simulink model "planning_control"  (R2020a)
settings: Solver=VariableStepAuto  StartTime=0.0  StopTime=40  RelTol=1e-3
undefined symbols (not defined in the file): aubr, tablebr, vubr
libraries: simulink x6, Solver_SF x2
settings Model: Creator=czj  LastModifiedBy=czj

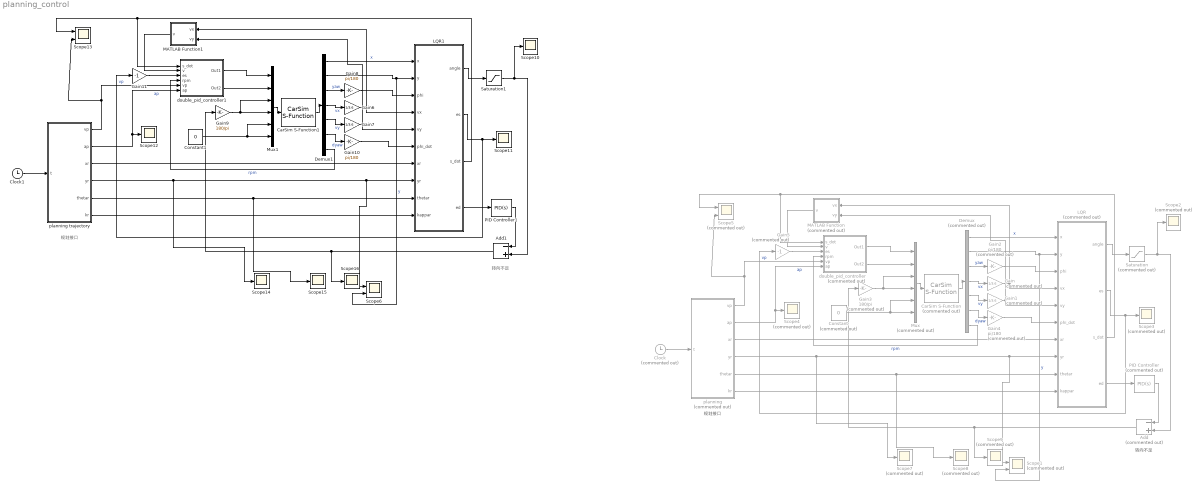
== system planning_control ==
  note: 规划接口
  note: 转向不足
  note: 规划接口
  note: 转向不足
  Add : Sum  Commented=on  Inputs=-+
  Add1 : Sum  Inputs=-+
  CarSim S-Function : Solver_SF/CarSim S-Function  Priority=1  Commented=on  SIMFILE=simfile.sim  Run_RTs=off  vs_state_ind=Run  StopMode_ind=Vehicle Model
  CarSim S-Function1 : Solver_SF/CarSim S-Function  Priority=1  SIMFILE=simfile.sim  Run_RTs=off  vs_state_ind=Run  StopMode_ind=Vehicle Model
  Clock : Clock  Commented=on
  Clock1 : Clock
  Constant : Constant  Commented=on  Value=0
  Constant1 : Constant  Value=0
  Demux : Demux  Commented=on  Outputs=7
  Demux1 : Demux  Outputs=7
  Gain : Gain  Commented=on  Gain=1/3.6
  Gain1 : Gain  Commented=on  Gain=1/3.6
  Gain10 : Gain  Gain=pi/180
  Gain11 : Gain  Gain=-1
  Gain2 : Gain  Commented=on  Gain=pi/180
  Gain3 : Gain  Commented=on  Gain=180/pi
  Gain4 : Gain  Commented=on  Gain=pi/180
  Gain5 : Gain  Commented=on  Gain=-1
  Gain6 : Gain  Gain=1/3.6
  Gain7 : Gain  Gain=1/3.6
  Gain8 : Gain  Gain=pi/180
  Gain9 : Gain  Gain=180/pi
  LQR : Subsystem  Commented=on
  LQR1 : Subsystem
  MATLAB Function : MATLAB Function  Commented=on  TreatAsAtomicUnit=on
  MATLAB Function1 : MATLAB Function  TreatAsAtomicUnit=on
  Mux : Mux  Commented=on  Inputs=6
  Mux1 : Mux  Inputs=6
  PID Controller : simulink/Continuous/PID Controller  Commented=on  Controller=PID  Form=Parallel  TimeDomain=Continuous-time  UseExternalTs=off  SampleTime=-1  IntegratorMethod=Forward Euler  FilterMethod=Forward Euler  ControllerParametersSource=internal  P=0  I=0  D=0  UseFilter=on  N=100  TunerSelectOption=Transfer Function Based (PID Tuner App)  InitialConditionSource=internal  InitialConditionForIntegrator=0  InitialConditionForFilter=0  DifferentiatorICPrevScaledInput=0  ExternalReset=none  TrackingMode=off  Kt=1  LimitOutput=off  UpperSaturationLimit=inf  LowerSaturationLimit=-inf  LinearizeAsGain=on  AntiWindupMode=none  Kb=1  POutMin=[]  POutMax=[]  IOutMin=[]  IOutMax=[]  DOutMin=[]  DOutMax=[]  NOutMin=[]  NOutMax=[]  SumOutMin=[]  SumOutMax=[]  SaturationOutMin=[]  SaturationOutMax=[]  PParamMin=[]  PParamMax=[]  IParamMin=[]  IParamMax=[]  DParamMin=[]  DParamMax=[]  NParamMin=[]  NParamMax=[]  KbParamMin=[]  KbParamMax=[]  KtParamMin=[]  KtParamMax=[]  KbOutMin=[]  KbOutMax=[]  KtOutMin=[]  KtOutMax=[]  IntegratorOutMin=[]  IntegratorOutMax=[]  FilterOutMin=[]  FilterOutMax=[]  SumI1OutMin=[]  SumI1OutMax=[]  SumI2OutMin=[]  SumI2OutMax=[]  SumI3OutMin=[]  SumI3OutMax=[]  SumI4OutMin=[]  SumI4OutMax=[]  SumDOutMin=[]  SumDOutMax=[]  DifferentiatorOutMin=[]  DifferentiatorOutMax=[]  FilterDiffOutCoefMin=[]  FilterDiffOutCoefMax=[]  ReciprocalOutMin=[]  ReciprocalOutMax=[]  SumDenOutMin=[]  SumDenOutMax=[]  SumNumOutMin=[]  SumNumOutMax=[]  DivideOutMin=[]  DivideOutMax=[]  UdiffTsProdOutMin=[]  UdiffTsProdOutMax=[]  NTsProdOutMin=[]  NTsProdOutMax=[]  UintegralTsProdOutMin=[]  UintegralTsProdOutMax=[]  UngainTsProdOutMin=[]  UngainTsProdOutMax=[]  IntegratorContinuousStateAttributes=''  IntegratorStateMustResolveToSignalObject=off  IntegratorRTWStateStorageClass=Auto  FilterContinuousStateAttributes=''  FilterStateMustResolveToSignalObject=off  FilterRTWStateStorageClass=Auto  ParallelPVariant=InternalParameters  IdealPVariant=Disabled  IVariant=InternalParameters  DVariant=InternalParameters  IntegratorVariant=Continuous  SatVariant=Disabled  AWVariant=Passthrough  PCopyVariant=Disabled  TRVariant=Disabled  FdbkBlocksVariant=Forward  IdealPFdbkVariant=Disabled  SatFdbkVariant=Disabled  DerivativeFilterVariant=ContFilter  NVariant=InternalParameters  NCopyVariant=Disabled  FilterICVariant=InternalICsFilter  IntegratorICVariant=InternalICs  ExternalResetVariant=Disabled  TRSumVariant=Passthrough  SumFdbkVariant=Disabled  SumVariant=Sum_PID  TsampFilterVariant=InternalTs  TsampNgainVariant=Passthrough  TsampIntegralVariant=Passthrough
  PID Controller1 : simulink/Continuous/PID Controller  Controller=PID  Form=Parallel  TimeDomain=Continuous-time  UseExternalTs=off  SampleTime=-1  IntegratorMethod=Forward Euler  FilterMethod=Forward Euler  ControllerParametersSource=internal  P=0  I=0  D=0  UseFilter=on  N=100  TunerSelectOption=Transfer Function Based (PID Tuner App)  InitialConditionSource=internal  InitialConditionForIntegrator=0  InitialConditionForFilter=0  DifferentiatorICPrevScaledInput=0  ExternalReset=none  TrackingMode=off  Kt=1  LimitOutput=off  UpperSaturationLimit=inf  LowerSaturationLimit=-inf  LinearizeAsGain=on  AntiWindupMode=none  Kb=1  POutMin=[]  POutMax=[]  IOutMin=[]  IOutMax=[]  DOutMin=[]  DOutMax=[]  NOutMin=[]  NOutMax=[]  SumOutMin=[]  SumOutMax=[]  SaturationOutMin=[]  SaturationOutMax=[]  PParamMin=[]  PParamMax=[]  IParamMin=[]  IParamMax=[]  DParamMin=[]  DParamMax=[]  NParamMin=[]  NParamMax=[]  KbParamMin=[]  KbParamMax=[]  KtParamMin=[]  KtParamMax=[]  KbOutMin=[]  KbOutMax=[]  KtOutMin=[]  KtOutMax=[]  IntegratorOutMin=[]  IntegratorOutMax=[]  FilterOutMin=[]  FilterOutMax=[]  SumI1OutMin=[]  SumI1OutMax=[]  SumI2OutMin=[]  SumI2OutMax=[]  SumI3OutMin=[]  SumI3OutMax=[]  SumI4OutMin=[]  SumI4OutMax=[]  SumDOutMin=[]  SumDOutMax=[]  DifferentiatorOutMin=[]  DifferentiatorOutMax=[]  FilterDiffOutCoefMin=[]  FilterDiffOutCoefMax=[]  ReciprocalOutMin=[]  ReciprocalOutMax=[]  SumDenOutMin=[]  SumDenOutMax=[]  SumNumOutMin=[]  SumNumOutMax=[]  DivideOutMin=[]  DivideOutMax=[]  UdiffTsProdOutMin=[]  UdiffTsProdOutMax=[]  NTsProdOutMin=[]  NTsProdOutMax=[]  UintegralTsProdOutMin=[]  UintegralTsProdOutMax=[]  UngainTsProdOutMin=[]  UngainTsProdOutMax=[]  IntegratorContinuousStateAttributes=''  IntegratorStateMustResolveToSignalObject=off  IntegratorRTWStateStorageClass=Auto  FilterContinuousStateAttributes=''  FilterStateMustResolveToSignalObject=off  FilterRTWStateStorageClass=Auto  ParallelPVariant=InternalParameters  IdealPVariant=Disabled  IVariant=InternalParameters  DVariant=InternalParameters  IntegratorVariant=Continuous  SatVariant=Disabled  AWVariant=Passthrough  PCopyVariant=Disabled  TRVariant=Disabled  FdbkBlocksVariant=Forward  IdealPFdbkVariant=Disabled  SatFdbkVariant=Disabled  DerivativeFilterVariant=ContFilter  NVariant=InternalParameters  NCopyVariant=Disabled  FilterICVariant=InternalICsFilter  IntegratorICVariant=InternalICs  ExternalResetVariant=Disabled  TRSumVariant=Passthrough  SumFdbkVariant=Disabled  SumVariant=Sum_PID  TsampFilterVariant=InternalTs  TsampNgainVariant=Passthrough  TsampIntegralVariant=Passthrough
  Saturation : Saturate  Commented=on  UpperLimit=1  LowerLimit=-1
  Saturation1 : Saturate  UpperLimit=1  LowerLimit=-1
  Scope1 : Scope  Commented=on  NumInputPorts=2
  Scope{10..12,14..16} (6 alike) : Scope
  Scope13 : Scope  NumInputPorts=2
  Scope{2..4,7..9} (6 alike) : Scope  Commented=on
  Scope5 : Scope  Commented=on  NumInputPorts=2
  Scope6 : Scope  NumInputPorts=2
  double_pid_controller : Subsystem  Commented=on
  double_pid_controller1 : Subsystem
  planning : MATLAB Function  Commented=on  TreatAsAtomicUnit=on
  planning trajectory : MATLAB Function  TreatAsAtomicUnit=on
  wires:
  CarSim S-Function/1 -> Demux/1
  PID Controller/1 -> Add/1
  LQR/3(s_dot) -> double_pid_controller/1(s_dot), Scope5/1
  Add/1 -> Scope9/1, Gain3/1
  Gain3/1 -> Mux/4, Mux/3
  Saturation/1 -> Scope2/1, Add/2
  planning/6(kr) -> LQR/10(kappar)
  LQR/2(es) -> Scope3/1, Gain5/1
  LQR/4(ed) -> PID Controller/1
  double_pid_controller/2(Out2) -> Mux/2
  Constant/1 -> Mux/5, Mux/6
  planning/2(ap) -> Scope4/1, double_pid_controller/6(ap)  "ap"
  Demux/3 -> Gain2/1  "yaw"
  Gain/1 -> MATLAB Function/1(vx), LQR/4(vx)
  Gain4/1 -> LQR/6(phi_dot)
  planning/3(xr) -> LQR/7(xr)
  Demux/6 -> Gain4/1  "dyaw"
  Mux/1 -> CarSim S-Function/1
  Gain5/1 -> double_pid_controller/3(es)
  Demux/5 -> Gain1/1  "vy"
  Demux/2 -> Scope1/2, LQR/2(y)  "y"
  double_pid_controller/1(Out1) -> Mux/1
  planning/5(thetar) -> Scope8/1, LQR/9(thetar)
  LQR/1(angle) -> Saturation/1
  planning/1(vp) -> Scope5/2, double_pid_controller/5(vp)  "vp"
  Gain1/1 -> MATLAB Function/2(vy), LQR/5(vy)
  Demux/7 -> double_pid_controller/4(rpm)  "rpm"
  Demux/1 -> LQR/1(x)  "x"
  Clock/1 -> planning/1(t)
  planning/4(yr) -> Scope7/1, Scope1/1, LQR/8(yr)
  MATLAB Function/1(v) -> double_pid_controller/2(v)
  Demux/4 -> Gain/1  "vx"
  Gain2/1 -> LQR/3(phi)
  CarSim S-Function1/1 -> Demux1/1
  PID Controller1/1 -> Add1/1
  LQR1/3(s_dot) -> double_pid_controller1/1(s_dot), Scope13/1
  Add1/1 -> Scope16/1, Gain9/1
  Gain9/1 -> Mux1/4, Mux1/3
  Saturation1/1 -> Scope10/1, Add1/2
  planning trajectory/6(kr) -> LQR1/10(kappar)
  LQR1/2(es) -> Scope11/1, Gain11/1
  LQR1/4(ed) -> PID Controller1/1
  double_pid_controller1/2(Out2) -> Mux1/2
  Constant1/1 -> Mux1/5, Mux1/6
  planning trajectory/2(ap) -> Scope12/1, double_pid_controller1/6(ap)  "ap"
  Demux1/3 -> Gain8/1  "yaw"
  Gain6/1 -> MATLAB Function1/1(vx), LQR1/4(vx)
  Gain10/1 -> LQR1/6(phi_dot)
  planning trajectory/3(xr) -> LQR1/7(xr)
  Demux1/6 -> Gain10/1  "dyaw"
  Mux1/1 -> CarSim S-Function1/1
  Gain11/1 -> double_pid_controller1/3(es)
  Demux1/5 -> Gain7/1  "vy"
  Demux1/2 -> Scope6/2, LQR1/2(y)  "y"
  double_pid_controller1/1(Out1) -> Mux1/1
  planning trajectory/5(thetar) -> Scope15/1, LQR1/9(thetar)
  LQR1/1(angle) -> Saturation1/1
  planning trajectory/1(vp) -> Scope13/2, double_pid_controller1/5(vp)  "vp"
  Gain7/1 -> MATLAB Function1/2(vy), LQR1/5(vy)
  Demux1/7 -> double_pid_controller1/4(rpm)  "rpm"
  Demux1/1 -> LQR1/1(x)  "x"
  Clock1/1 -> planning trajectory/1(t)
  planning trajectory/4(yr) -> Scope14/1, Scope6/1, LQR1/8(yr)
  MATLAB Function1/1(v) -> double_pid_controller1/2(v)
  Demux1/4 -> Gain6/1  "vx"
  Gain8/1 -> LQR1/3(phi)

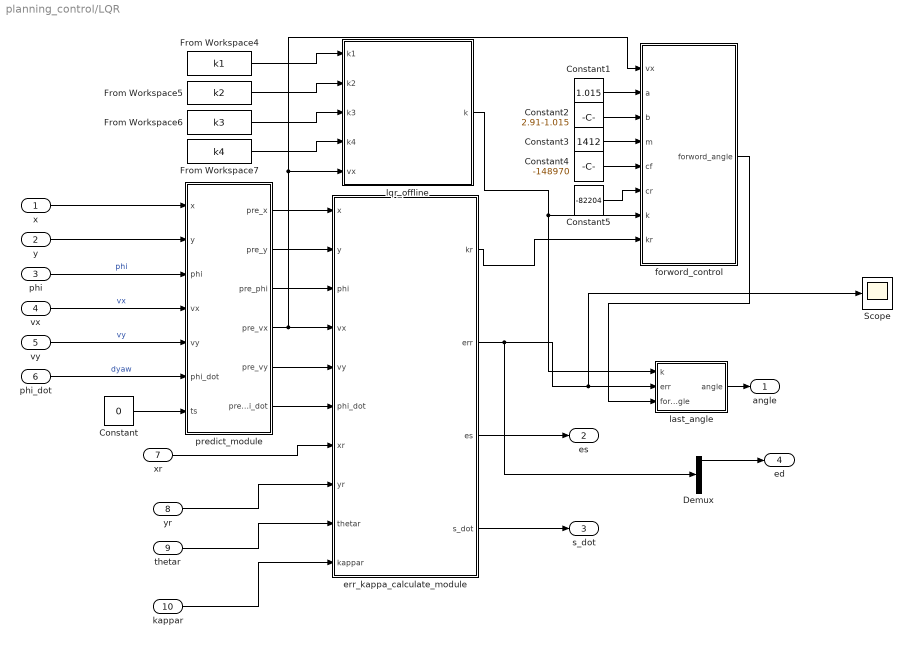
== system planning_control/LQR ==
  x : Inport
  y : Inport  Port=2
  phi : Inport  Port=3
  vx : Inport  Port=4
  vy : Inport  Port=5
  phi_dot : Inport  Port=6
  xr : Inport  Port=7
  yr : Inport  Port=8
  thetar : Inport  Port=9
  kappar : Inport  Port=10
  Constant : Constant  Value=0
  Constant1 : Constant  Value=1.015
  Constant2 : Constant  Value=2.91-1.015
  Constant3 : Constant  Value=1412
  Constant4 : Constant  Value=-148970
  Constant5 : Constant  Value=-82204
  Demux : Demux
  From Workspace4 : FromWorkspace  VariableName=k1
  From Workspace5 : FromWorkspace  VariableName=k2
  From Workspace6 : FromWorkspace  VariableName=k3
  From Workspace7 : FromWorkspace  VariableName=k4
  Scope : Scope
  err_kappa_calculate_module : MATLAB Function  TreatAsAtomicUnit=on
  forword_control : MATLAB Function  TreatAsAtomicUnit=on
  last_angle : MATLAB Function  TreatAsAtomicUnit=on
  lqr_offline : MATLAB Function  TreatAsAtomicUnit=on
  predict_module : MATLAB Function  TreatAsAtomicUnit=on
  angle : Outport  VectorParamsAs1DForOutWhenUnconnected=off
  es : Outport  Port=2  VectorParamsAs1DForOutWhenUnconnected=off
  s_dot : Outport  Port=3  VectorParamsAs1DForOutWhenUnconnected=off
  ed : Outport  Port=4  VectorParamsAs1DForOutWhenUnconnected=off
  wires:
  From Workspace7/1 -> lqr_offline/4(k4)
  vy/1 -> predict_module/5(vy)  "vy"
  From Workspace6/1 -> lqr_offline/3(k3)
  x/1 -> predict_module/1(x)
  lqr_offline/1(k) -> last_angle/1(k), forword_control/7(k)
  predict_module/2(pre_y) -> err_kappa_calculate_module/2(y)
  err_kappa_calculate_module/1(kr) -> forword_control/8(kr)
  forword_control/1(forword_angle) -> last_angle/3(forword_angle)
  predict_module/4(pre_vx) -> lqr_offline/5(vx), forword_control/1(vx), err_kappa_calculate_module/4(vx)
  phi_dot/1 -> predict_module/6(phi_dot)  "dyaw"
  last_angle/1(angle) -> angle/1
  From Workspace5/1 -> lqr_offline/2(k2)
  vx/1 -> predict_module/4(vx)  "vx"
  y/1 -> predict_module/2(y)
  phi/1 -> predict_module/3(phi)  "phi"
  Constant/1 -> predict_module/7(ts)
  From Workspace4/1 -> lqr_offline/1(k1)
  predict_module/1(pre_x) -> err_kappa_calculate_module/1(x)
  predict_module/5(pre_vy) -> err_kappa_calculate_module/5(vy)
  predict_module/6(pre_phi_dot) -> err_kappa_calculate_module/6(phi_dot)
  predict_module/3(pre_phi) -> err_kappa_calculate_module/3(phi)
  Constant1/1 -> forword_control/2(a)
  Constant2/1 -> forword_control/3(b)
  Constant3/1 -> forword_control/4(m)
  Constant4/1 -> forword_control/5(cf)
  xr/1 -> err_kappa_calculate_module/7(xr)
  yr/1 -> err_kappa_calculate_module/8(yr)
  thetar/1 -> err_kappa_calculate_module/9(thetar)
  kappar/1 -> err_kappa_calculate_module/10(kappar)
  err_kappa_calculate_module/3(es) -> es/1
  err_kappa_calculate_module/4(s_dot) -> s_dot/1
  Constant5/1 -> forword_control/6(cr)
  Demux/1 -> ed/1
  err_kappa_calculate_module/2(err) -> Demux/1, Scope/1, last_angle/2(err)

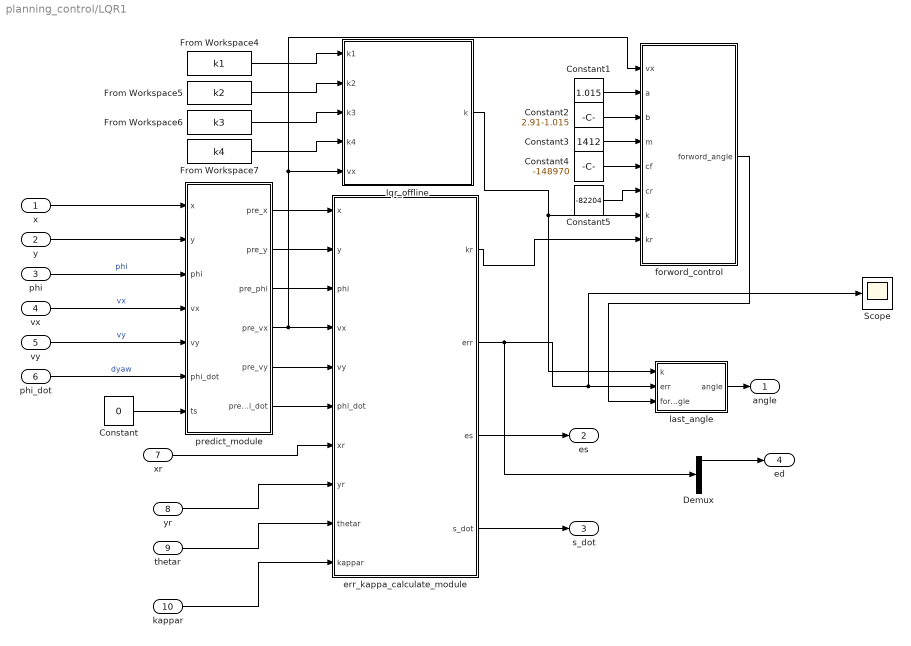
== system planning_control/LQR1 ==
  x : Inport
  y : Inport  Port=2
  phi : Inport  Port=3
  vx : Inport  Port=4
  vy : Inport  Port=5
  phi_dot : Inport  Port=6
  xr : Inport  Port=7
  yr : Inport  Port=8
  thetar : Inport  Port=9
  kappar : Inport  Port=10
  Constant : Constant  Value=0
  Constant1 : Constant  Value=1.015
  Constant2 : Constant  Value=2.91-1.015
  Constant3 : Constant  Value=1412
  Constant4 : Constant  Value=-148970
  Constant5 : Constant  Value=-82204
  Demux : Demux
  From Workspace4 : FromWorkspace  VariableName=k1
  From Workspace5 : FromWorkspace  VariableName=k2
  From Workspace6 : FromWorkspace  VariableName=k3
  From Workspace7 : FromWorkspace  VariableName=k4
  Scope : Scope
  err_kappa_calculate_module : MATLAB Function  TreatAsAtomicUnit=on
  forword_control : MATLAB Function  TreatAsAtomicUnit=on
  last_angle : MATLAB Function  TreatAsAtomicUnit=on
  lqr_offline : MATLAB Function  TreatAsAtomicUnit=on
  predict_module : MATLAB Function  TreatAsAtomicUnit=on
  angle : Outport  VectorParamsAs1DForOutWhenUnconnected=off
  es : Outport  Port=2  VectorParamsAs1DForOutWhenUnconnected=off
  s_dot : Outport  Port=3  VectorParamsAs1DForOutWhenUnconnected=off
  ed : Outport  Port=4  VectorParamsAs1DForOutWhenUnconnected=off
  wires:
  From Workspace7/1 -> lqr_offline/4(k4)
  vy/1 -> predict_module/5(vy)  "vy"
  From Workspace6/1 -> lqr_offline/3(k3)
  x/1 -> predict_module/1(x)
  lqr_offline/1(k) -> last_angle/1(k), forword_control/7(k)
  predict_module/2(pre_y) -> err_kappa_calculate_module/2(y)
  err_kappa_calculate_module/1(kr) -> forword_control/8(kr)
  forword_control/1(forword_angle) -> last_angle/3(forword_angle)
  predict_module/4(pre_vx) -> lqr_offline/5(vx), forword_control/1(vx), err_kappa_calculate_module/4(vx)
  phi_dot/1 -> predict_module/6(phi_dot)  "dyaw"
  last_angle/1(angle) -> angle/1
  From Workspace5/1 -> lqr_offline/2(k2)
  vx/1 -> predict_module/4(vx)  "vx"
  y/1 -> predict_module/2(y)
  phi/1 -> predict_module/3(phi)  "phi"
  Constant/1 -> predict_module/7(ts)
  From Workspace4/1 -> lqr_offline/1(k1)
  predict_module/1(pre_x) -> err_kappa_calculate_module/1(x)
  predict_module/5(pre_vy) -> err_kappa_calculate_module/5(vy)
  predict_module/6(pre_phi_dot) -> err_kappa_calculate_module/6(phi_dot)
  predict_module/3(pre_phi) -> err_kappa_calculate_module/3(phi)
  Constant1/1 -> forword_control/2(a)
  Constant2/1 -> forword_control/3(b)
  Constant3/1 -> forword_control/4(m)
  Constant4/1 -> forword_control/5(cf)
  xr/1 -> err_kappa_calculate_module/7(xr)
  yr/1 -> err_kappa_calculate_module/8(yr)
  thetar/1 -> err_kappa_calculate_module/9(thetar)
  kappar/1 -> err_kappa_calculate_module/10(kappar)
  err_kappa_calculate_module/3(es) -> es/1
  err_kappa_calculate_module/4(s_dot) -> s_dot/1
  Constant5/1 -> forword_control/6(cr)
  Demux/1 -> ed/1
  err_kappa_calculate_module/2(err) -> Demux/1, Scope/1, last_angle/2(err)

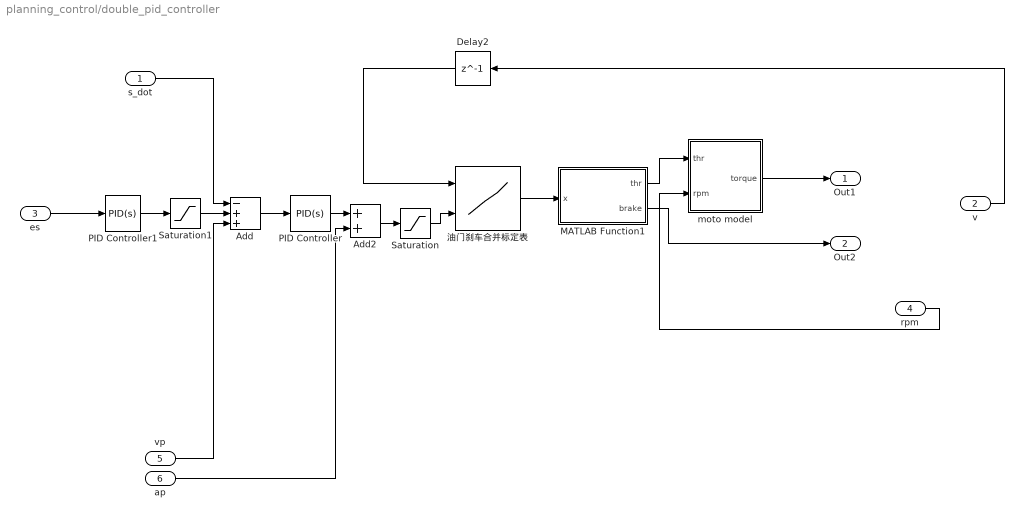
== system planning_control/double_pid_controller ==
  s_dot : Inport
  v : Inport  Port=2
  es : Inport  Port=3
  rpm : Inport  Port=4
  vp : Inport  Port=5
  ap : Inport  Port=6
  Add : Sum  Inputs=-++
  Add2 : Sum
  Delay2 : Delay  DelayLength=1
  MATLAB Function1 : MATLAB Function  TreatAsAtomicUnit=on
  PID Controller : simulink/Continuous/PID Controller  Controller=PID  Form=Parallel  TimeDomain=Continuous-time  UseExternalTs=off  SampleTime=-1  IntegratorMethod=Forward Euler  FilterMethod=Forward Euler  ControllerParametersSource=internal  P=3  I=0  D=0.1  UseFilter=on  N=30  TunerSelectOption=Transfer Function Based (PID Tuner App)  InitialConditionSource=internal  InitialConditionForIntegrator=0  InitialConditionForFilter=0  DifferentiatorICPrevScaledInput=0  ExternalReset=none  TrackingMode=off  Kt=1  LimitOutput=off  UpperSaturationLimit=inf  LowerSaturationLimit=-inf  LinearizeAsGain=on  AntiWindupMode=none  Kb=1  POutMin=[]  POutMax=[]  IOutMin=[]  IOutMax=[]  DOutMin=[]  DOutMax=[]  NOutMin=[]  NOutMax=[]  SumOutMin=[]  SumOutMax=[]  SaturationOutMin=[]  SaturationOutMax=[]  PParamMin=[]  PParamMax=[]  IParamMin=[]  IParamMax=[]  DParamMin=[]  DParamMax=[]  NParamMin=[]  NParamMax=[]  KbParamMin=[]  KbParamMax=[]  KtParamMin=[]  KtParamMax=[]  KbOutMin=[]  KbOutMax=[]  KtOutMin=[]  KtOutMax=[]  IntegratorOutMin=[]  IntegratorOutMax=[]  FilterOutMin=[]  FilterOutMax=[]  SumI1OutMin=[]  SumI1OutMax=[]  SumI2OutMin=[]  SumI2OutMax=[]  SumI3OutMin=[]  SumI3OutMax=[]  SumI4OutMin=[]  SumI4OutMax=[]  SumDOutMin=[]  SumDOutMax=[]  DifferentiatorOutMin=[]  DifferentiatorOutMax=[]  FilterDiffOutCoefMin=[]  FilterDiffOutCoefMax=[]  ReciprocalOutMin=[]  ReciprocalOutMax=[]  SumDenOutMin=[]  SumDenOutMax=[]  SumNumOutMin=[]  SumNumOutMax=[]  DivideOutMin=[]  DivideOutMax=[]  UdiffTsProdOutMin=[]  UdiffTsProdOutMax=[]  NTsProdOutMin=[]  NTsProdOutMax=[]  UintegralTsProdOutMin=[]  UintegralTsProdOutMax=[]  UngainTsProdOutMin=[]  UngainTsProdOutMax=[]  IntegratorContinuousStateAttributes=''  IntegratorStateMustResolveToSignalObject=off  IntegratorRTWStateStorageClass=Auto  FilterContinuousStateAttributes=''  FilterStateMustResolveToSignalObject=off  FilterRTWStateStorageClass=Auto  ParallelPVariant=InternalParameters  IdealPVariant=Disabled  IVariant=InternalParameters  DVariant=InternalParameters  IntegratorVariant=Continuous  SatVariant=Disabled  AWVariant=Passthrough  PCopyVariant=Disabled  TRVariant=Disabled  FdbkBlocksVariant=Forward  IdealPFdbkVariant=Disabled  SatFdbkVariant=Disabled  DerivativeFilterVariant=ContFilter  NVariant=InternalParameters  NCopyVariant=Disabled  FilterICVariant=InternalICsFilter  IntegratorICVariant=InternalICs  ExternalResetVariant=Disabled  TRSumVariant=Passthrough  SumFdbkVariant=Disabled  SumVariant=Sum_PID  TsampFilterVariant=InternalTs  TsampNgainVariant=Passthrough  TsampIntegralVariant=Passthrough
  PID Controller1 : simulink/Continuous/PID Controller  Controller=PID  Form=Parallel  TimeDomain=Continuous-time  UseExternalTs=off  SampleTime=-1  IntegratorMethod=Forward Euler  FilterMethod=Forward Euler  ControllerParametersSource=internal  P=3  I=0  D=0.1  UseFilter=on  N=30  TunerSelectOption=Transfer Function Based (PID Tuner App)  InitialConditionSource=internal  InitialConditionForIntegrator=0  InitialConditionForFilter=0  DifferentiatorICPrevScaledInput=0  ExternalReset=none  TrackingMode=off  Kt=1  LimitOutput=off  UpperSaturationLimit=inf  LowerSaturationLimit=-inf  LinearizeAsGain=on  AntiWindupMode=none  Kb=1  POutMin=[]  POutMax=[]  IOutMin=[]  IOutMax=[]  DOutMin=[]  DOutMax=[]  NOutMin=[]  NOutMax=[]  SumOutMin=[]  SumOutMax=[]  SaturationOutMin=[]  SaturationOutMax=[]  PParamMin=[]  PParamMax=[]  IParamMin=[]  IParamMax=[]  DParamMin=[]  DParamMax=[]  NParamMin=[]  NParamMax=[]  KbParamMin=[]  KbParamMax=[]  KtParamMin=[]  KtParamMax=[]  KbOutMin=[]  KbOutMax=[]  KtOutMin=[]  KtOutMax=[]  IntegratorOutMin=[]  IntegratorOutMax=[]  FilterOutMin=[]  FilterOutMax=[]  SumI1OutMin=[]  SumI1OutMax=[]  SumI2OutMin=[]  SumI2OutMax=[]  SumI3OutMin=[]  SumI3OutMax=[]  SumI4OutMin=[]  SumI4OutMax=[]  SumDOutMin=[]  SumDOutMax=[]  DifferentiatorOutMin=[]  DifferentiatorOutMax=[]  FilterDiffOutCoefMin=[]  FilterDiffOutCoefMax=[]  ReciprocalOutMin=[]  ReciprocalOutMax=[]  SumDenOutMin=[]  SumDenOutMax=[]  SumNumOutMin=[]  SumNumOutMax=[]  DivideOutMin=[]  DivideOutMax=[]  UdiffTsProdOutMin=[]  UdiffTsProdOutMax=[]  NTsProdOutMin=[]  NTsProdOutMax=[]  UintegralTsProdOutMin=[]  UintegralTsProdOutMax=[]  UngainTsProdOutMin=[]  UngainTsProdOutMax=[]  IntegratorContinuousStateAttributes=''  IntegratorStateMustResolveToSignalObject=off  IntegratorRTWStateStorageClass=Auto  FilterContinuousStateAttributes=''  FilterStateMustResolveToSignalObject=off  FilterRTWStateStorageClass=Auto  ParallelPVariant=InternalParameters  IdealPVariant=Disabled  IVariant=InternalParameters  DVariant=InternalParameters  IntegratorVariant=Continuous  SatVariant=Disabled  AWVariant=Passthrough  PCopyVariant=Disabled  TRVariant=Disabled  FdbkBlocksVariant=Forward  IdealPFdbkVariant=Disabled  SatFdbkVariant=Disabled  DerivativeFilterVariant=ContFilter  NVariant=InternalParameters  NCopyVariant=Disabled  FilterICVariant=InternalICsFilter  IntegratorICVariant=InternalICs  ExternalResetVariant=Disabled  TRSumVariant=Passthrough  SumFdbkVariant=Disabled  SumVariant=Sum_PID  TsampFilterVariant=InternalTs  TsampNgainVariant=Passthrough  TsampIntegralVariant=Passthrough
  Saturation : Saturate  UpperLimit=5  LowerLimit=-8
  Saturation1 : Saturate  UpperLimit=10  LowerLimit=-10
  moto model : MATLAB Function  TreatAsAtomicUnit=on
  油门刹车合并标定表 : Lookup_n-D  BreakpointsForDimension1=vubr  BreakpointsForDimension2=aubr  Table=tablebr  InternalRulePriority=Speed  RndMeth=Simplest  InputSameDT=on
  Out1 : Outport  VectorParamsAs1DForOutWhenUnconnected=off
  Out2 : Outport  Port=2  VectorParamsAs1DForOutWhenUnconnected=off
  wires:
  v/1 -> Delay2/1
  ap/1 -> Add2/2
  Add2/1 -> Saturation/1
  Saturation/1 -> 油门刹车合并标定表/2
  Delay2/1 -> 油门刹车合并标定表/1
  油门刹车合并标定表/1 -> MATLAB Function1/1(x)
  Add/1 -> PID Controller/1
  PID Controller/1 -> Add2/1
  MATLAB Function1/1(thr) -> moto model/1(thr)
  PID Controller1/1 -> Saturation1/1
  moto model/1(torque) -> Out1/1
  MATLAB Function1/2(brake) -> Out2/1
  vp/1 -> Add/3
  es/1 -> PID Controller1/1
  s_dot/1 -> Add/1
  rpm/1 -> moto model/2(rpm)
  Saturation1/1 -> Add/2

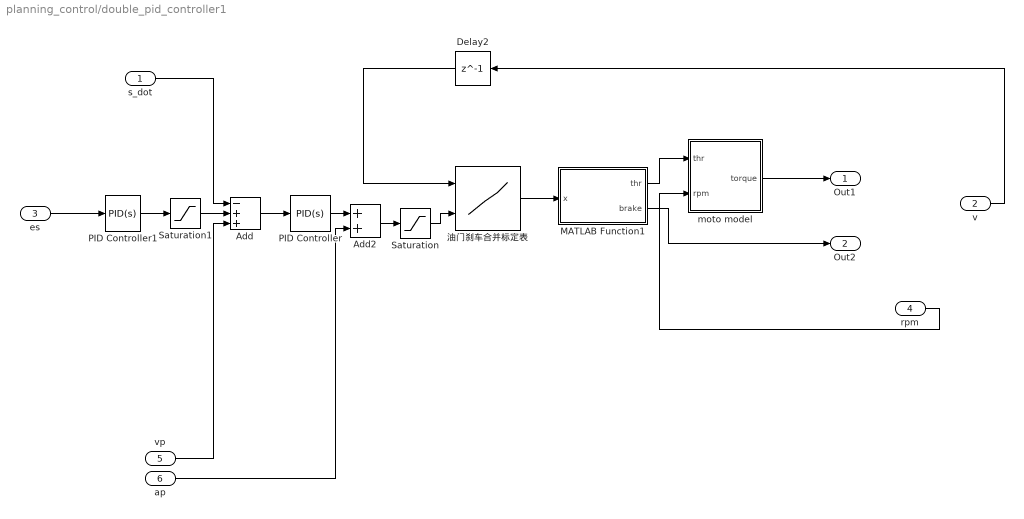
== system planning_control/double_pid_controller1 ==
  s_dot : Inport
  v : Inport  Port=2
  es : Inport  Port=3
  rpm : Inport  Port=4
  vp : Inport  Port=5
  ap : Inport  Port=6
  Add : Sum  Inputs=-++
  Add2 : Sum
  Delay2 : Delay  DelayLength=1
  MATLAB Function1 : MATLAB Function  TreatAsAtomicUnit=on
  PID Controller : simulink/Continuous/PID Controller  Controller=PID  Form=Parallel  TimeDomain=Continuous-time  UseExternalTs=off  SampleTime=-1  IntegratorMethod=Forward Euler  FilterMethod=Forward Euler  ControllerParametersSource=internal  P=3  I=0  D=0.1  UseFilter=on  N=30  TunerSelectOption=Transfer Function Based (PID Tuner App)  InitialConditionSource=internal  InitialConditionForIntegrator=0  InitialConditionForFilter=0  DifferentiatorICPrevScaledInput=0  ExternalReset=none  TrackingMode=off  Kt=1  LimitOutput=off  UpperSaturationLimit=inf  LowerSaturationLimit=-inf  LinearizeAsGain=on  AntiWindupMode=none  Kb=1  POutMin=[]  POutMax=[]  IOutMin=[]  IOutMax=[]  DOutMin=[]  DOutMax=[]  NOutMin=[]  NOutMax=[]  SumOutMin=[]  SumOutMax=[]  SaturationOutMin=[]  SaturationOutMax=[]  PParamMin=[]  PParamMax=[]  IParamMin=[]  IParamMax=[]  DParamMin=[]  DParamMax=[]  NParamMin=[]  NParamMax=[]  KbParamMin=[]  KbParamMax=[]  KtParamMin=[]  KtParamMax=[]  KbOutMin=[]  KbOutMax=[]  KtOutMin=[]  KtOutMax=[]  IntegratorOutMin=[]  IntegratorOutMax=[]  FilterOutMin=[]  FilterOutMax=[]  SumI1OutMin=[]  SumI1OutMax=[]  SumI2OutMin=[]  SumI2OutMax=[]  SumI3OutMin=[]  SumI3OutMax=[]  SumI4OutMin=[]  SumI4OutMax=[]  SumDOutMin=[]  SumDOutMax=[]  DifferentiatorOutMin=[]  DifferentiatorOutMax=[]  FilterDiffOutCoefMin=[]  FilterDiffOutCoefMax=[]  ReciprocalOutMin=[]  ReciprocalOutMax=[]  SumDenOutMin=[]  SumDenOutMax=[]  SumNumOutMin=[]  SumNumOutMax=[]  DivideOutMin=[]  DivideOutMax=[]  UdiffTsProdOutMin=[]  UdiffTsProdOutMax=[]  NTsProdOutMin=[]  NTsProdOutMax=[]  UintegralTsProdOutMin=[]  UintegralTsProdOutMax=[]  UngainTsProdOutMin=[]  UngainTsProdOutMax=[]  IntegratorContinuousStateAttributes=''  IntegratorStateMustResolveToSignalObject=off  IntegratorRTWStateStorageClass=Auto  FilterContinuousStateAttributes=''  FilterStateMustResolveToSignalObject=off  FilterRTWStateStorageClass=Auto  ParallelPVariant=InternalParameters  IdealPVariant=Disabled  IVariant=InternalParameters  DVariant=InternalParameters  IntegratorVariant=Continuous  SatVariant=Disabled  AWVariant=Passthrough  PCopyVariant=Disabled  TRVariant=Disabled  FdbkBlocksVariant=Forward  IdealPFdbkVariant=Disabled  SatFdbkVariant=Disabled  DerivativeFilterVariant=ContFilter  NVariant=InternalParameters  NCopyVariant=Disabled  FilterICVariant=InternalICsFilter  IntegratorICVariant=InternalICs  ExternalResetVariant=Disabled  TRSumVariant=Passthrough  SumFdbkVariant=Disabled  SumVariant=Sum_PID  TsampFilterVariant=InternalTs  TsampNgainVariant=Passthrough  TsampIntegralVariant=Passthrough
  PID Controller1 : simulink/Continuous/PID Controller  Controller=PID  Form=Parallel  TimeDomain=Continuous-time  UseExternalTs=off  SampleTime=-1  IntegratorMethod=Forward Euler  FilterMethod=Forward Euler  ControllerParametersSource=internal  P=3  I=0  D=0.1  UseFilter=on  N=30  TunerSelectOption=Transfer Function Based (PID Tuner App)  InitialConditionSource=internal  InitialConditionForIntegrator=0  InitialConditionForFilter=0  DifferentiatorICPrevScaledInput=0  ExternalReset=none  TrackingMode=off  Kt=1  LimitOutput=off  UpperSaturationLimit=inf  LowerSaturationLimit=-inf  LinearizeAsGain=on  AntiWindupMode=none  Kb=1  POutMin=[]  POutMax=[]  IOutMin=[]  IOutMax=[]  DOutMin=[]  DOutMax=[]  NOutMin=[]  NOutMax=[]  SumOutMin=[]  SumOutMax=[]  SaturationOutMin=[]  SaturationOutMax=[]  PParamMin=[]  PParamMax=[]  IParamMin=[]  IParamMax=[]  DParamMin=[]  DParamMax=[]  NParamMin=[]  NParamMax=[]  KbParamMin=[]  KbParamMax=[]  KtParamMin=[]  KtParamMax=[]  KbOutMin=[]  KbOutMax=[]  KtOutMin=[]  KtOutMax=[]  IntegratorOutMin=[]  IntegratorOutMax=[]  FilterOutMin=[]  FilterOutMax=[]  SumI1OutMin=[]  SumI1OutMax=[]  SumI2OutMin=[]  SumI2OutMax=[]  SumI3OutMin=[]  SumI3OutMax=[]  SumI4OutMin=[]  SumI4OutMax=[]  SumDOutMin=[]  SumDOutMax=[]  DifferentiatorOutMin=[]  DifferentiatorOutMax=[]  FilterDiffOutCoefMin=[]  FilterDiffOutCoefMax=[]  ReciprocalOutMin=[]  ReciprocalOutMax=[]  SumDenOutMin=[]  SumDenOutMax=[]  SumNumOutMin=[]  SumNumOutMax=[]  DivideOutMin=[]  DivideOutMax=[]  UdiffTsProdOutMin=[]  UdiffTsProdOutMax=[]  NTsProdOutMin=[]  NTsProdOutMax=[]  UintegralTsProdOutMin=[]  UintegralTsProdOutMax=[]  UngainTsProdOutMin=[]  UngainTsProdOutMax=[]  IntegratorContinuousStateAttributes=''  IntegratorStateMustResolveToSignalObject=off  IntegratorRTWStateStorageClass=Auto  FilterContinuousStateAttributes=''  FilterStateMustResolveToSignalObject=off  FilterRTWStateStorageClass=Auto  ParallelPVariant=InternalParameters  IdealPVariant=Disabled  IVariant=InternalParameters  DVariant=InternalParameters  IntegratorVariant=Continuous  SatVariant=Disabled  AWVariant=Passthrough  PCopyVariant=Disabled  TRVariant=Disabled  FdbkBlocksVariant=Forward  IdealPFdbkVariant=Disabled  SatFdbkVariant=Disabled  DerivativeFilterVariant=ContFilter  NVariant=InternalParameters  NCopyVariant=Disabled  FilterICVariant=InternalICsFilter  IntegratorICVariant=InternalICs  ExternalResetVariant=Disabled  TRSumVariant=Passthrough  SumFdbkVariant=Disabled  SumVariant=Sum_PID  TsampFilterVariant=InternalTs  TsampNgainVariant=Passthrough  TsampIntegralVariant=Passthrough
  Saturation : Saturate  UpperLimit=5  LowerLimit=-8
  Saturation1 : Saturate  UpperLimit=10  LowerLimit=-10
  moto model : MATLAB Function  TreatAsAtomicUnit=on
  油门刹车合并标定表 : Lookup_n-D  BreakpointsForDimension1=vubr  BreakpointsForDimension2=aubr  Table=tablebr  InternalRulePriority=Speed  RndMeth=Simplest  InputSameDT=on
  Out1 : Outport  VectorParamsAs1DForOutWhenUnconnected=off
  Out2 : Outport  Port=2  VectorParamsAs1DForOutWhenUnconnected=off
  wires:
  v/1 -> Delay2/1
  ap/1 -> Add2/2
  Add2/1 -> Saturation/1
  Saturation/1 -> 油门刹车合并标定表/2
  Delay2/1 -> 油门刹车合并标定表/1
  油门刹车合并标定表/1 -> MATLAB Function1/1(x)
  Add/1 -> PID Controller/1
  PID Controller/1 -> Add2/1
  MATLAB Function1/1(thr) -> moto model/1(thr)
  PID Controller1/1 -> Saturation1/1
  moto model/1(torque) -> Out1/1
  MATLAB Function1/2(brake) -> Out2/1
  vp/1 -> Add/3
  es/1 -> PID Controller1/1
  s_dot/1 -> Add/1
  rpm/1 -> moto model/2(rpm)
  Saturation1/1 -> Add/2

== matlab function planning_control/LQR/predict_module ==
  data: x input; pre_x output; y input; phi input; vx input; vy input; phi_dot input; ts input; pre_y output; pre_phi output; pre_vx output; pre_vy output; pre_phi_dot output
function [pre_x,pre_y,pre_phi,pre_vx,pre_vy,pre_phi_dot] = fcn(x,y,phi,vx,vy,phi_dot,ts)
    pre_x=x+vx*ts*cos(phi)-vy*ts*sin(phi);
    pre_y=y+vy*ts*cos(phi)+vx*ts*sin(phi);
    pre_phi=phi+phi_dot*ts;
    pre_vx=vx;
    pre_vy=vy;
    pre_phi_dot=phi_dot;
end

== matlab function planning_control/LQR1/err_kappa_calculate_module ==
  data: x input; kr output; y input; phi input; vx input; vy input; phi_dot input; xr input; yr input; thetar input; kappar input; err output; es output; s_dot output
function [kr,err,es,s_dot] = fcn(x,y,phi,vx,vy,phi_dot,xr,yr,thetar,kappar)
    
    tor=[cos(thetar);sin(thetar)];
    nor=[-sin(thetar);cos(thetar)];
    d_err=[x-xr;y-yr];
    ed=nor'*d_err;
    es=tor'*d_err;
    %projection_point_thetar=thetar(dmin);%apollo
    projection_point_thetar=thetar+kappar*es;
    ed_dot=vy*cos(phi-projection_point_thetar)+vx*sin(phi-projection_point_thetar);
    %%%%%%%%%
    ephi=sin(phi-projection_point_thetar);
    %%%%%%%%%
    ss_dot=vx*cos(phi-projection_point_thetar)-vy*sin(phi-projection_point_thetar);
    s_dot=ss_dot/(1-kappar*ed);
    ephi_dot=phi_dot-kappar*s_dot;
    kr=kappar;
    err=[ed;ed_dot;ephi;ephi_dot];
    
    
    
    
    
    
    
    
    
    
    
    


end

== matlab function planning_control/LQR1/forword_control ==
  data: vx input; a input; forword_angle output; b input; m input; cf input; cr input; k input; kr input
function forword_angle = fcn(vx,a,b,m,cf,cr,k,kr)
    forword_angle=kr*(a+b-b*k(3)-(m*vx*vx/(a+b))*((b/cf)+(a/cr)*k(3)-(a/cr)));
end

== matlab function planning_control/LQR1/last_angle ==
  data: k input; angle output; err input; forword_angle input
function angle = fcn(k,err,forword_angle)

    angle=-k*err+forword_angle;
end

== matlab function planning_control/LQR1/lqr_offline ==
  data: k1 input; k output; k2 input; k3 input; k4 input; vx input
function k  = fcn(k1,k2,k3,k4,vx)
    if abs(vx)<0.01
        k=[0,0,0,0];
    else
        index=round(vx/0.01);
        k=[k1(index),k2(index),k3(index),k4(index)];
    end
end

== matlab function planning_control/LQR1/predict_module ==
  data: x input; pre_x output; y input; phi input; vx input; vy input; phi_dot input; ts input; pre_y output; pre_phi output; pre_vx output; pre_vy output; pre_phi_dot output
function [pre_x,pre_y,pre_phi,pre_vx,pre_vy,pre_phi_dot] = fcn(x,y,phi,vx,vy,phi_dot,ts)
    pre_x=x+vx*ts*cos(phi)-vy*ts*sin(phi);
    pre_y=y+vy*ts*cos(phi)+vx*ts*sin(phi);
    pre_phi=phi+phi_dot*ts;
    pre_vx=vx;
    pre_vy=vy;
    pre_phi_dot=phi_dot;
end

== matlab function planning_control/double_pid_controller/MATLAB Function1 ==
  data: x input; thr output; brake output
function [thr,brake] = fcn(x)
    %正数代表油门，负数代表刹车
    %不允许同时踩油门和刹车
    if x>=0
        thr=x;
        brake=0;
    else
        thr=0;
        brake=-x;
    end

== matlab function planning_control/MATLAB Function1 ==
  data: vx input; v output; vy input
function v = fcn(vx,vy)
    v=sqrt(vx^2+vy^2);

== matlab function planning_control/double_pid_controller1/MATLAB Function1 ==
  data: x input; thr output; brake output
function [thr,brake] = fcn(x)
    %正数代表油门，负数代表刹车
    %不允许同时踩油门和刹车
    if x>=0
        thr=x;
        brake=0;
    else
        thr=0;
        brake=-x;
    end

== matlab function planning_control/double_pid_controller1/moto model ==
  data: thr input; torque output; rpm input
function torque = fcn(thr,rpm)
Tmax=380*thr;
    if (rpm<=4523)
        torque=Tmax;
    else
        torque=Tmax*4523/rpm;
    end
end

== matlab function planning_control/planning trajectory ==
  data: vp output; ap output; t input; xr output; yr output; thetar output; kr output
function [vp,ap,xr,yr,thetar,kr] = fcn(t)
    dx=100;
    dy=10;
    T=30;
    xstart=[0,0,0];
    xend=[dx,0,0];
    ystart=[0,0,0];
    yend=[dy,0,0];
    a=zeros(1,6);
    b=zeros(1,6);
    
    a(1)=xstart(1);
    a(2)=xstart(2);
    a(3)=xstart(3)/2;
    A1=[T^3,T^4,T^5;
        3*T^2,4*T^3,5*T^4;
        6*T,12*T^2,20*T^3];
    B1=[xend(1)-a(1)-a(2)*T-a(3)*T^2;
        xend(2)-a(2)-2*a(3)*T;
        xend(3)-2*a(3)];
    xs=inv(A1)*B1;
    a(4)=xs(1);
    a(5)=xs(2);
    a(6)=xs(3);
    b(1)=ystart(1);
    b(2)=ystart(2);
    b(3)=ystart(3)/2;
    A2=[dx^3,dx^4,dx^5;
        3*dx^2,4*dx^3,5*dx^4;
        6*dx,12*dx^2,20*dx^3];
    B2=[yend(1)-b(1)-b(2)*dx-b(3)*dx^2;
        yend(2)-b(2)-2*b(3)*dx;
        yend(3)-2*b(3)];
    ys=inv(A2)*B2;
    b(4)=ys(1);
    b(5)=ys(2);
    b(6)=ys(3);
    xr=a(1)+a(2)*t+a(3)*t^2+a(4)*t^3+a(5)*t^4+a(6)*t^5;
    yr=b(1)+b(2)*xr+b(3)*xr^2+b(4)*xr^3+b(5)*xr^4+b(6)*xr^5;
    xr_dot=a(2)+2*a(3)*t+3*a(4)*t^2+4*a(5)*t^3+5*a(6)*t^4;
    yr_dx=b(2)+2*b(3)*xr+3*b(4)*xr^2+4*b(5)*xr^3+5*b(6)*xr^4;
    yr_dot=yr_dx*xr_dot;
    thetar=atan(yr_dx);
    xr_dot2=2*a(3)+6*a(4)*t+12*a(5)*t^2+20*a(6)*t^3;
    yr_dx2=2*b(3)+6*b(4)*xr+12*b(5)*xr^2+20*b(6)*xr^3;
    yr_dot2=yr_dx2*xr_dot^2+yr_dx*xr_dot2;
    kr=yr_dx2/((1+yr_dx^2)^1.5);
    vp=sqrt(xr_dot^2+yr_dot^2);
    if xr_dot2>=0
        ap=sqrt(xr_dot2^2+yr_dot2^2);
    else
        ap=-sqrt(xr_dot2^2+yr_dot2^2);
    end

== matlab function planning_control/double_pid_controller/moto model ==
  data: thr input; torque output; rpm input
function torque = fcn(thr,rpm)
Tmax=380*thr;
    if (rpm<=4523)
        torque=Tmax;
    else
        torque=Tmax*4523/rpm;
    end
end

== matlab function planning_control/planning ==
  data: vp output; ap output; t input; xr output; yr output; thetar output; kr output
function [vp,ap,xr,yr,thetar,kr] = fcn(t)
    dx=100;
    dy=10;
    T=30;
    xstart=[0,0,0];
    xend=[dx,0,0];
    ystart=[0,0,0];
    yend=[dy,0,0];
    a=zeros(1,6);
    b=zeros(1,6);
    
    a(1)=xstart(1);
    a(2)=xstart(2);
    a(3)=xstart(3)/2;
    A1=[T^3,T^4,T^5;
        3*T^2,4*T^3,5*T^4;
        6*T,12*T^2,20*T^3];
    B1=[xend(1)-a(1)-a(2)*T-a(3)*T^2;
        xend(2)-a(2)-2*a(3)*T;
        xend(3)-2*a(3)];
    xs=inv(A1)*B1;
    a(4)=xs(1);
    a(5)=xs(2);
    a(6)=xs(3);
    b(1)=ystart(1);
    b(2)=ystart(2);
    b(3)=ystart(3)/2;
    A2=[dx^3,dx^4,dx^5;
        3*dx^2,4*dx^3,5*dx^4;
        6*dx,12*dx^2,20*dx^3];
    B2=[yend(1)-b(1)-b(2)*dx-b(3)*dx^2;
        yend(2)-b(2)-2*b(3)*dx;
        yend(3)-2*b(3)];
    ys=inv(A2)*B2;
    b(4)=ys(1);
    b(5)=ys(2);
    b(6)=ys(3);
    xr=a(1)+a(2)*t+a(3)*t^2+a(4)*t^3+a(5)*t^4+a(6)*t^5;
    yr=b(1)+b(2)*xr+b(3)*xr^2+b(4)*xr^3+b(5)*xr^4+b(6)*xr^5;
    xr_dot=a(2)+2*a(3)*t+3*a(4)*t^2+4*a(5)*t^3+5*a(6)*t^4;
    yr_dx=b(2)+2*b(3)*xr+3*b(4)*xr^2+4*b(5)*xr^3+5*b(6)*xr^4;
    yr_dot=yr_dx*xr_dot;
    thetar=atan(yr_dx);
    xr_dot2=2*a(3)+6*a(4)*t+12*a(5)*t^2+20*a(6)*t^3;
    yr_dx2=2*b(3)+6*b(4)*xr+12*b(5)*xr^2+20*b(6)*xr^3;
    yr_dot2=yr_dx2*xr_dot^2+yr_dx*xr_dot2;
    kr=yr_dx2/((1+yr_dx^2)^1.5);
    vp=sqrt(xr_dot^2+yr_dot^2);
    if xr_dot2>=0
        ap=sqrt(xr_dot2^2+yr_dot2^2);
    else
        ap=-sqrt(xr_dot2^2+yr_dot2^2);
    end

== matlab function planning_control/MATLAB Function ==
  data: vx input; v output; vy input
function v = fcn(vx,vy)
    v=sqrt(vx^2+vy^2);

== matlab function planning_control/LQR/err_kappa_calculate_module ==
  data: x input; kr output; y input; phi input; vx input; vy input; phi_dot input; xr input; yr input; thetar input; kappar input; err output; es output; s_dot output
function [kr,err,es,s_dot] = fcn(x,y,phi,vx,vy,phi_dot,xr,yr,thetar,kappar)
    
    tor=[cos(thetar);sin(thetar)];
    nor=[-sin(thetar);cos(thetar)];
    d_err=[x-xr;y-yr];
    ed=nor'*d_err;
    es=tor'*d_err;
    %projection_point_thetar=thetar(dmin);%apollo
    projection_point_thetar=thetar+kappar*es;
    ed_dot=vy*cos(phi-projection_point_thetar)+vx*sin(phi-projection_point_thetar);
    %%%%%%%%%
    ephi=sin(phi-projection_point_thetar);
    %%%%%%%%%
    ss_dot=vx*cos(phi-projection_point_thetar)-vy*sin(phi-projection_point_thetar);
    s_dot=ss_dot/(1-kappar*ed);
    ephi_dot=phi_dot-kappar*s_dot;
    kr=kappar;
    err=[ed;ed_dot;ephi;ephi_dot];
    
    
    
    
    
    
    
    
    
    
    
    


end

== matlab function planning_control/LQR/forword_control ==
  data: vx input; a input; forword_angle output; b input; m input; cf input; cr input; k input; kr input
function forword_angle = fcn(vx,a,b,m,cf,cr,k,kr)
    forword_angle=kr*(a+b-b*k(3)-(m*vx*vx/(a+b))*((b/cf)+(a/cr)*k(3)-(a/cr)));
end

== matlab function planning_control/LQR/last_angle ==
  data: k input; angle output; err input; forword_angle input
function angle = fcn(k,err,forword_angle)

    angle=-k*err+forword_angle;
end

== matlab function planning_control/LQR/lqr_offline ==
  data: k1 input; k output; k2 input; k3 input; k4 input; vx input
function k  = fcn(k1,k2,k3,k4,vx)
    if abs(vx)<0.01
        k=[0,0,0,0];
    else
        index=round(vx/0.01);
        k=[k1(index),k2(index),k3(index),k4(index)];
    end
end
